simulink model "iWalkerHokuyoModel"  (R2014a)
settings: Solver=ode3  StartTime=0.0  StopTime=Inf  RelTol=1e-3
StartFcn:
  | localAddEventListener('iWalkerHokuyoModel');
libraries: iWalkerLib x8
settings Model: Creator=Brian  LastModifiedBy=Brian
settings OptimizationCC: BlockReduction=off

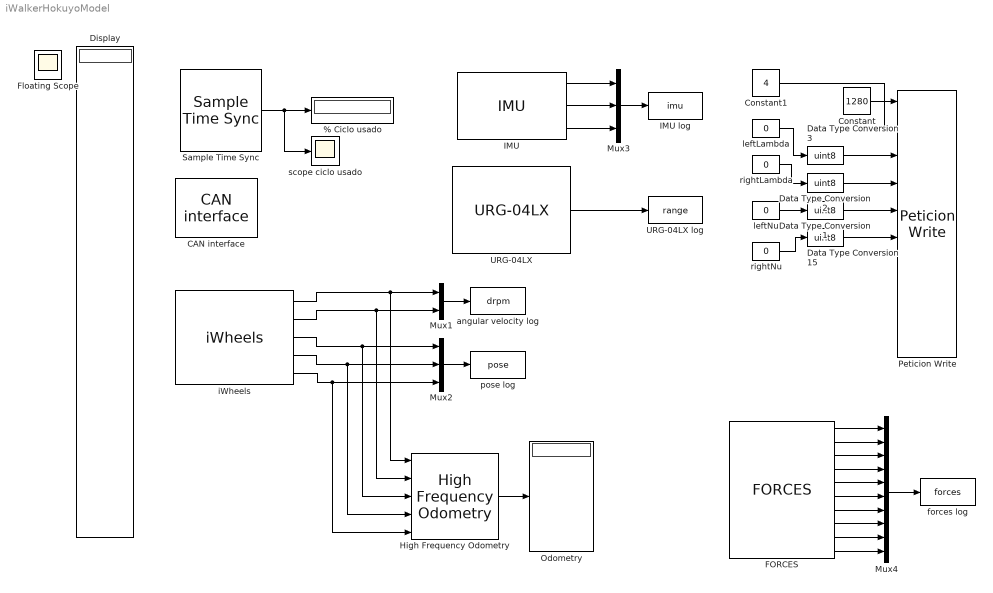
== system iWalkerHokuyoModel ==
  % Ciclo usado : Display
      settings: Decimation=100
  CAN interface : iWalkerLib/CAN interface
  Constant : Constant  Value=1280  SampleTime=1
  Constant1 : Constant  Value=4  SampleTime=1
  Data Type Conversion{1..3,15} (4 alike) : DataTypeConversion  OutDataTypeStr=uint8  ConvertRealWorld=Stored Integer (SI)
  Display : Display
      settings: Floating=on
  FORCES : iWalkerLib/FORCES  SampleTime=0.1
  Floating Scope : Scope
      settings: Floating=on  SaveName=ScopeData2
  High Frequency Odometry : iWalkerLib/High Frequency Odometry
  IMU : iWalkerLib/IMU  SampleTime=0.1
  IMU log : ToWorkspace  VariableName=imu  SaveFormat=Timeseries  SampleTime=-1
  Mux1 : Mux  Inputs=2
  Mux2 : Mux  Inputs=3
  Mux3 : Mux  Inputs=3
  Mux4 : Mux  Inputs=10
  Odometry : Display
  Peticion Write : iWalkerLib/Peticion Write  Priority=0
  Sample Time Sync : iWalkerLib/Sample Time Sync  Priority=8  SampleTime=0.1
  URG-04LX : iWalkerLib/URG-04LX  COM=7  SampleTime=0.3  Verbose=off
  URG-04LX log : ToWorkspace  VariableName=range  SaveFormat=Timeseries  SampleTime=-1
  angular velocity log : ToWorkspace  VariableName=drpm  SaveFormat=Timeseries  SampleTime=-1
  forces log : ToWorkspace  VariableName=forces  SaveFormat=Timeseries  SampleTime=-1
  iWheels : iWalkerLib/iWheels  SampleTime=0.1
  leftLambda : Constant  Value=0  SampleTime=1
  leftNu : Constant  Value=0  SampleTime=1
  pose log : ToWorkspace  VariableName=pose  SaveFormat=Timeseries  SampleTime=-1
  rightLambda : Constant  Value=0  SampleTime=1
  rightNu : Constant  Value=0  SampleTime=1
  scope ciclo usado : Scope
      settings: TimeRange=0.7489177489177488  YMin=0  YMax=250
  wires:
  URG-04LX/1 -> URG-04LX log/1
  Sample Time Sync/1 -> scope ciclo usado/1, % Ciclo usado/1
  Mux1/1 -> angular velocity log/1
  iWheels/1 -> High Frequency Odometry/1, Mux1/1
  iWheels/2 -> High Frequency Odometry/2, Mux1/2
  iWheels/3 -> High Frequency Odometry/3, Mux2/1
  iWheels/4 -> High Frequency Odometry/4, Mux2/2
  iWheels/5 -> High Frequency Odometry/5, Mux2/3
  Mux2/1 -> pose log/1
  IMU/1 -> Mux3/1
  IMU/2 -> Mux3/2
  Mux3/1 -> IMU log/1
  FORCES/1 -> Mux4/1
  FORCES/2 -> Mux4/2
  FORCES/3 -> Mux4/3
  FORCES/4 -> Mux4/4
  FORCES/5 -> Mux4/5
  FORCES/6 -> Mux4/6
  FORCES/7 -> Mux4/7
  FORCES/8 -> Mux4/8
  FORCES/9 -> Mux4/9
  FORCES/10 -> Mux4/10
  Mux4/1 -> forces log/1
  Constant/1 -> Peticion Write/1
  Constant1/1 -> Peticion Write/2
  rightNu/1 -> Data Type Conversion15/1
  Data Type Conversion15/1 -> Peticion Write/6
  leftNu/1 -> Data Type Conversion1/1
  Data Type Conversion1/1 -> Peticion Write/5
  rightLambda/1 -> Data Type Conversion2/1
  Data Type Conversion2/1 -> Peticion Write/4
  leftLambda/1 -> Data Type Conversion3/1
  Data Type Conversion3/1 -> Peticion Write/3
  IMU/3 -> Mux3/3
  High Frequency Odometry/1 -> Odometry/1
